simulink model "P5p5c"  (Simulink 8.9)
settings: Solver=ode45  StartTime=0.0  StopTime=400  RelTol=1e-3  EnableMultiTasking=on
values from neighbouring files (symbols this model uses):
  Kpd = 0.84    [P5p5c.m]    (also in P5p5d.m; P5p5e.m)
  Td = T    (= 72.52)    [P5p5c.m]    (also in P5p5d.m; P5p5e.m)
  Tf = 8.36    [P5p5c.m]    (also in P5p5d.m; P5p5e.m)
  timeSample = 1/10    (= 0.1)    [P5p5c.m]    (also in P5p5d.m; P5p5e.m)
libraries: simulink x2, simulink_extras x2
settings Model: Creator=markh  LastModifiedBy=nicholao
settings DataIOCC: SignalLoggingName=sigsOut
settings OptimizationCC: InitFltsAndDblsToZero=on
settings DebuggingCC: SaveWithParameterizedLinksMsg=none  SignalResolutionControl=TryResolveAllWithWarning  MultiTaskDSMMsg=warning  MultiTaskCondExecSysMsg=none
settings HardwareCC: TargetUnknown=on
settings GRTTargetCC: TargetFcnLib=ansi_tfl_tmw.mat

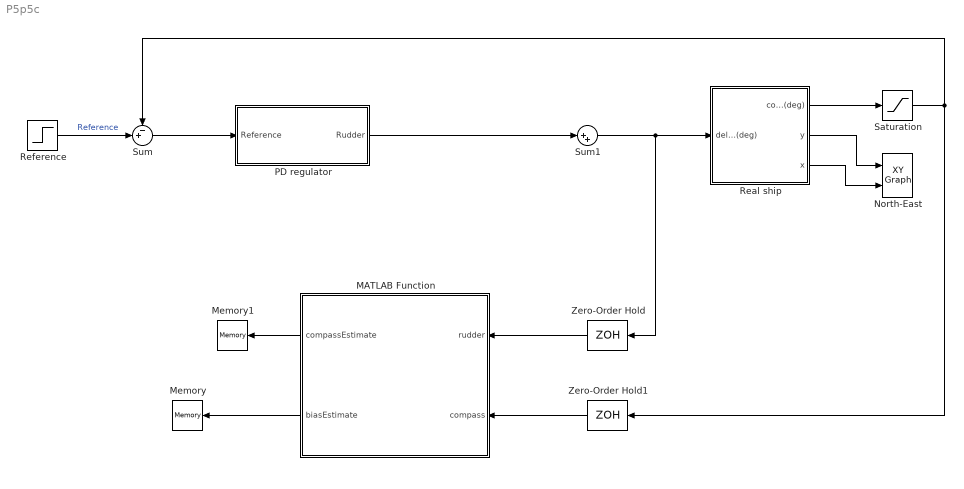
== system P5p5c ==
  MATLAB Function : MATLAB Function  TreatAsAtomicUnit=on
  Memory : Memory
  Memory1 : Memory
  North-East : simulink/Sinks/XY Graph  xmin=-5000  xmax=6000  ymin=-5000  ymax=5000  st=-1
  PD regulator : Subsystem
  Real ship : Subsystem  mask(Simple shipmodel for a cargo ship){noise=on, current=off, logic=off}
      mask prompts: noise "measurement noise"; logic "waves"
      mask help:
      | Measurement noise:
      | 	checked = noise on
      | 	unchecked = noise off
      |
      | Current:
      | 	checked = current on
      | 	unchecked = current off
      |
      | Waves:
      | 	checked = waves on
      | 	unchecked = waves off
      |
      | Author: Jørgen Spjøtvold, 9/10-2003
      | TTK 4115 Linear system theory.
      | Modified by Jostein Bakkeheim 26/10-2006
  Reference : Step  After=30  SampleTime=0
  Saturation : Saturate  UpperLimit=35  LowerLimit=-35
  Sum : Sum  Inputs=-+|
  Sum1 : Sum  Inputs=|++
  Zero-Order Hold : ZeroOrderHold  SampleTime=timeSample
  Zero-Order Hold1 : ZeroOrderHold  SampleTime=timeSample
  wires:
  Real ship/3(x) -> North-East/2
  Real ship/2(y) -> North-East/1
  Real ship/1(compass (deg)) -> Saturation/1
  Reference/1 -> Sum/2  "Reference"
  Zero-Order Hold/1 -> MATLAB Function/1(rudder)
  Zero-Order Hold1/1 -> MATLAB Function/2(compass)
  MATLAB Function/1(compassEstimate) -> Memory1/1
  MATLAB Function/2(biasEstimate) -> Memory/1
  Sum1/1 -> Zero-Order Hold/1, Real ship/1(delta (deg))
  Saturation/1 -> Zero-Order Hold1/1, Sum/1
  Sum/1 -> PD regulator/1(Reference)
  PD regulator/1(Rudder) -> Sum1/1

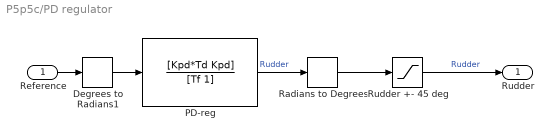
== system P5p5c/PD regulator ==
  Reference : Inport
  Degrees to Radians1 : simulink_extras/Transformations/Degrees to Radians
  PD-reg : TransferFcn  Numerator=[Kpd*Td Kpd]  Denominator=[Tf 1]
  Radians to Degrees : simulink_extras/Transformations/Radians to Degrees
  "Rudder +- 45 deg " : Saturate  UpperLimit=45  LowerLimit=-45
  Rudder : Outport
  wires:
  Degrees to Radians1/1 -> PD-reg/1
  "Rudder +- 45 deg "/1 -> Rudder/1  "Rudder"
  Reference/1 -> Degrees to Radians1/1
  PD-reg/1 -> Radians to Degrees/1  "Rudder"
  Radians to Degrees/1 -> "Rudder +- 45 deg "/1

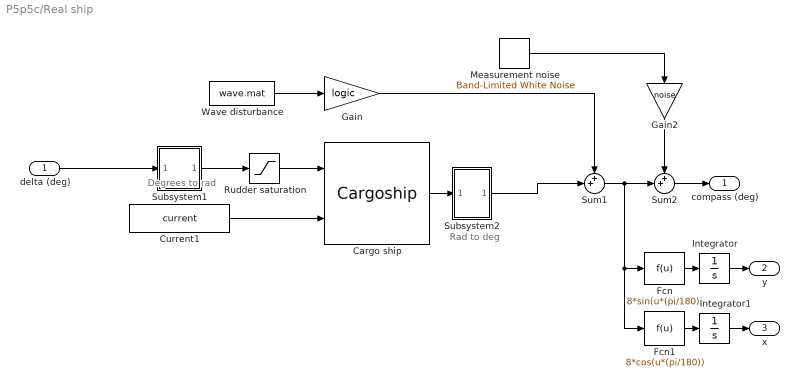
== system P5p5c/Real ship ==
  note: Degrees to rad
  note: Rad to deg
  delta (deg) : Inport
  Cargo ship : S-Function  FunctionName=Cargoship  SFunctionDeploymentMode=off  EnableBusSupport=off  mask(Cargo ship){}
      mask help:
      | S-function which simulates a cargo ship.
      |
      | Author: Jørgen Spjøtvold
      | 20.10-2003
      | Modified by Jostein Bakkeheim 27.10.2006
  Current1 : Constant  Value=current
  Fcn : Fcn  Expr=8*sin(u*(pi/180))
  Fcn1 : Fcn  Expr=8*cos(u*(pi/180))
  Gain : Gain  Gain=logic  SaturateOnIntegerOverflow=on  OutDataTypeStr=Inherit: Same as input  ParamDataTypeStr=Inherit: Same as input
  Gain2 : Gain  Gain=noise  SaturateOnIntegerOverflow=on  OutDataTypeStr=Inherit: Same as input  ParamDataTypeStr=Inherit: Same as input
  Integrator : Integrator
  Integrator1 : Integrator
  Measurement noise : simulink/Sources/Band-Limited White Noise  Cov=[0.001]  Ts=.5  seed=[23341]
  Rudder saturation : Saturate  UpperLimit=45*(pi/180)  LowerLimit=-45*(pi/180)
  Subsystem1 : Subsystem  mask(degrees to radians){}
      mask help: Converts degrees to radians
      mask Display: fprintf('D2R');
  Subsystem2 : Subsystem  mask(radians to degrees){}
      mask help: Converts radians to degrees
      mask Display: fprintf('R2D');
  Sum1 : Sum  Inputs=++|  SaturateOnIntegerOverflow=on
  Sum2 : Sum  Inputs=++|  SaturateOnIntegerOverflow=on
  Wave disturbance : FromFile  FileName=wave.mat  SampleTime=0
  compass (deg) : Outport
  y : Outport  Port=2
  x : Outport  Port=3
  wires:
  delta (deg)/1 -> Subsystem1/1(In1)
  Fcn/1 -> Integrator/1
  Integrator/1 -> y/1
  Fcn1/1 -> Integrator1/1
  Integrator1/1 -> x/1
  Wave disturbance/1 -> Gain/1
  Subsystem2/1(Out1) -> Sum1/2
  Sum1/1 -> Fcn/1, Fcn1/1, Sum2/2
  Cargo ship/1 -> Subsystem2/1(In1)
  Subsystem1/1(Out1) -> Rudder saturation/1
  Rudder saturation/1 -> Cargo ship/1
  Sum2/1 -> compass (deg)/1
  Measurement noise/1 -> Gain2/1
  Gain2/1 -> Sum2/1
  Current1/1 -> Cargo ship/2
  Gain/1 -> Sum1/1

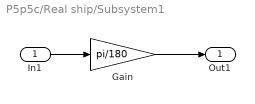
== system P5p5c/Real ship/Subsystem1 ==
  In1 : Inport
  Gain : Gain  Gain=pi/180  SaturateOnIntegerOverflow=on  OutDataTypeStr=Inherit: Same as input  ParamDataTypeStr=Inherit: Same as input
  Out1 : Outport
  wires:
  Gain/1 -> Out1/1
  In1/1 -> Gain/1

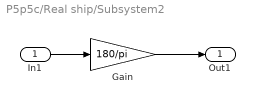
== system P5p5c/Real ship/Subsystem2 ==
  In1 : Inport
  Gain : Gain  Gain=180/pi  SaturateOnIntegerOverflow=on  OutDataTypeStr=Inherit: Same as input  ParamDataTypeStr=Inherit: Same as input
  Out1 : Outport
  wires:
  Gain/1 -> Out1/1
  In1/1 -> Gain/1

== matlab function MATLAB Function ==
  data: rudder input double; compassEstimate output double; compass input double; biasEstimate output double; dataStruct parameter double
function [compassEstimate, biasEstimate] = Kalman(rudder, compass, dataStruct)

persistent init_flag A B C E Q R P_ x_


if isempty(init_flag)
    % Initialization for system
    init_flag = 1;
    
    [A,B,C,E,Q,R,P_,x_] = deal(dataStruct.A, dataStruct.B, dataStruct.C, ...
                            dataStruct.E, dataStruct.Q, dataStruct.R,...
                            dataStruct.P_, dataStruct.x_);
end

I = eye(5);

K =  (P_*C')*inv((C*P_*C'+R));

x = x_ + K*(compass-C*x_);

P = (I-K*C)*P_*(I-K*C)'+K*R*K';

x_ = A*x + B*rudder;

P_ = A*P*A'+E*Q*E';

compassEstimate = x(3);
biasEstimate = x(5);
end
